simulink library "MuteControl"  (R2022b)
settings: Solver=VariableStepAuto  StartTime=0.0  StopTime=10.0  RelTol=1e-3
libraries: MuteControlBtc x1
settings Model: Creator=db1045444  LastModifiedBy=kl13806
settings SolverCC: AlgebraicLoopSolver=TrustRegion
settings DebuggingCC: UnconnectedInputMsg=warning  UnconnectedOutputMsg=warning  UnconnectedLineMsg=warning  SFMachineParentedDataDiag=warning
settings ModelReferenceCC: EnableRefExpFcnMdlSchedulingChecks=on
settings RTWCC: DLArmComputeVersion=19.05

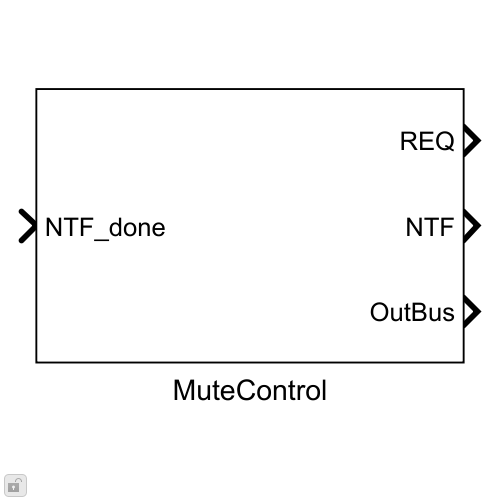
[thumbnail: Simulink's stored preview of the top-level diagram]
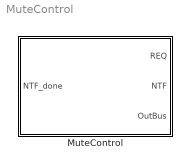
== system MuteControl ==
  MuteControl : Subsystem  mask(Bose MuteControl){}
      mask help: This component is to be used in conjunction with 1 or more instances of the MuteRamper block. There is no mask for this component. It provides the control layer for Mute processing via an RTC and tune variable, muteControlRampTime.
      mask init:
      | InnerLinkConfig = MuteControlConfig;
      mask Help: If this control block is being used in a "multi-instance" manner, i.e. it is contorlling two or more MuteRamper blocks, there is an additional step that must be done. The developer must add a function-triggered subsytem containing an AND logic gate, which will combine the notification completion signals of the multiple ramper instances. The output of this subsytem must then feed the NTF_done input of the MuteControl block.

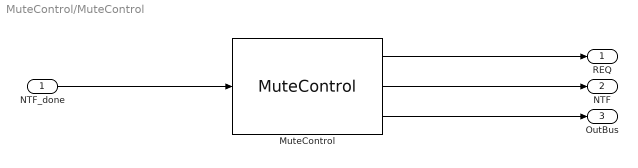
== system MuteControl/MuteControl ==
  NTF_done : Inport
  MuteControl : MuteControlBtc/MuteControl  Config=InnerLinkConfig  FeatureName=MuteControl
      settings: SourceProductName=Bose Blocklib
  REQ : Outport
  NTF : Outport  Port=2
  OutBus : Outport  Port=3
  wires:
  MuteControl/1 -> REQ/1
  MuteControl/2 -> NTF/1
  MuteControl/3 -> OutBus/1
  NTF_done/1 -> MuteControl/1
